simulink model "Boost_and_Two_Level_Inverter_IO"  (R2021b)
settings: Solver=ode3  StartTime=0.0  StopTime=inf  FixedStep=Ts  RelTol=1e-3
PostLoadFcn:
  | Boost_and_Two_Level_Inverter_param;
InitFcn:
  | Boost_and_Two_Level_Inverter_param;
undefined symbols (not defined in the file): arm1_g1, Boost2lvl_SFun, boost_I, Boost_PWM_Duty, Boost_PWM_Freq, boost_V, Boost_Vin, d9cbfad2d710, eHSx128_Gen4_Machines_IOConfig1, EX, fault_sw, Inv_BEMF_Ampl, Inv_PWM_CarrierFreq, Inv_PWM_ModulationIndex, Inv_PWM_Out, Inv_PWM_Phases, Inv_PWM_ShiftAngle, Ts, v1, VC707_2, vin, vsrc1, vsrc2, vsrc3
libraries: opal_lib x3, rtlab x3, rtio_opalrt_common x2, ehsSchematicEditorSourceLib x1, ehsFirmwareSelection x1
PreSaveFcn:
  | try, efsUpdateVersionAnnotation, end
settings Model: ARTEMISmethode_block_infos=$$__separator__$$  Creator=PYRobert  LastModifiedBy=ORTGRemotePC
settings SolverCC: AlgebraicLoopSolver=TrustRegion
settings DataIOCC: LimitDataPoints=on  SaveFormat=Array  SignalLoggingSaveFormat=ModelDataLogs  SaveOutput=off  SignalLogging=off  SaveTime=off  ReturnWorkspaceOutputs=off  SignalLoggingName=sigsOut
settings OptimizationCC: BlockReduction=off  OptimizeBlockIOStorage=off  BufferReuse=off  GlobalBufferReuse=off  ExpressionFolding=off  ExpressionDepthLimit=2147483647  LocalBlockOutputs=off  InitFltsAndDblsToZero=on  LifeSpan=inf  OptimizeDataStoreBuffers=off  BusAssignmentInplaceUpdate=off
settings DebuggingCC: SaveWithParameterizedLinksMsg=none  UnderspecifiedInitializationDetection=Classic  MergeDetectMultiDrivingBlocksExec=none  SignalResolutionControl=TryResolveAllWithWarning  InheritedTsInSrcMsg=none  MultiTaskDSMMsg=warning  MultiTaskCondExecSysMsg=none  ParameterOverflowMsg=none  FcnCallInpInsideContextMsg=warning  StateNameClashWarn=warning  SFUnexpectedBacktrackingDiag=warning  SFNoUnconditionalDefaultTransitionDiag=warning  SFExecutionAtInitializationDiag=none  SFMachineParentedDataDiag=warning  ArithmeticOperatorsInVariantConditions=warning
settings HardwareCC: ProdBitPerPointer=32  ProdBitPerSizeT=32  ProdBitPerPtrDiffT=32  ProdLargestAtomicFloat=None  ProdIntDivRoundTo=Undefined  ProdEndianess=Unspecified  ProdWordSize=32  ProdHWDeviceType=32-bit Generic  TargetBitPerPointer=64  TargetBitPerSizeT=64  TargetBitPerPtrDiffT=64  TargetLongLongMode=on  TargetIntDivRoundTo=Zero  TargetEndianess=LittleEndian  TargetWordSize=64  TargetHWDeviceType=MATLAB Host  ProdEqTarget=off
settings ModelReferenceCC: PropagateSignalLabelsOutOfModel=off
settings SFSimCC: SimUseLocalCustomCode=off  CustomCodeUndefinedFunction=UseInterfaceOnly
settings RTWCC: RTWUseLocalCustomCode=off
settings CodeAppCC: StateflowObjectComments=on
settings GRTTargetCC: TargetFcnLib=ansi_tfl_tmw.mat  TargetLangStandard=C89/C90 (ANSI)  CombineOutputUpdateFcns=off  GRTInterface=on
settings ConfigComp: CovMetricSettings=dw  CovSaveCumulativeToWorkspaceVar=on  CovSaveSingleToWorkspaceVar=on  CovExternalEMLEnable=off  CovSFcnEnable=off
settings SimscapeCC: SimscapeNormalizeSystem=off

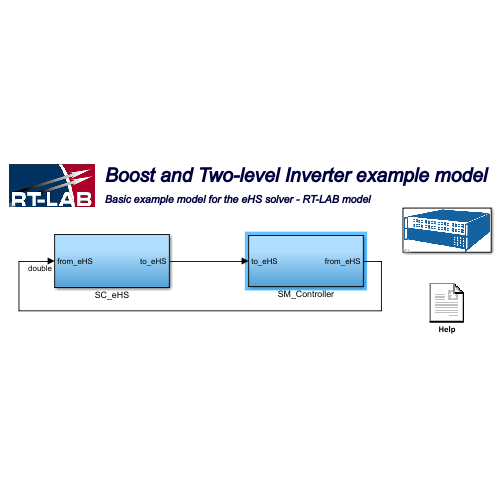
[thumbnail: Simulink's stored preview of the top-level diagram]
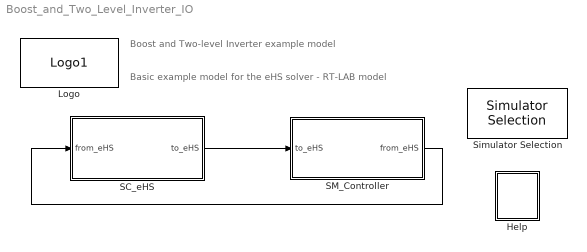
== system Boost_and_Two_Level_Inverter_IO ==
  note: Boost and Two-level Inverter example model
  note: Basic example model for the eHS solver - RT-LAB model
  Help : Subsystem  mask(OpDoc){docfile=\Docs\html\Examples\Boost-and-Two-Level-Inverter---S-Function---eHS-Gen4.html}
      mask init:
      | %patch([1,1,0,0,.8,1],[.8,0,0,1,1,.8],[.8 .8 .8]);
      | %patch([.15 .78 .78 .15 .15],[.8 .8 .83 .83 .8],[.9 .9 .9]);
      | %patch([.15 .78 .78 .15 .15],[.7 .7 .73 .73 .8],[.9 .9 .9]);
      | %patch([.15 .78 .78 .15 .15],[.6 .6 .63 .63 .6],[.9 .9 .9]);
      | %patch([.15 .78 .78 .15 .15],[.5 .5 .53 .53 .5],[.9 .9 .9]);
      | %patch([.15 .78 .78 .15 .15],[.4 .4 .43 .43 .4],[.9 .9 .9]);
      settings: OpenFcn=efsHelp_cb(gcb);
      mask Display: image(imread('opdoc.bmp'))
  Logo : opal_lib/Logo1  vide=[]
  SC_eHS : Subsystem
  SM_Controller : Subsystem
  Simulator Selection : ehsFirmwareSelection/Simulator Selection  wChassisSelection=OP5707  eHSType=SE
  wires:
  SC_eHS/1(to_eHS) -> SM_Controller/1(to_eHS)
  SM_Controller/1(from_eHS) -> SC_eHS/1(from_eHS)

== system Boost_and_Two_Level_Inverter_IO/Help ==

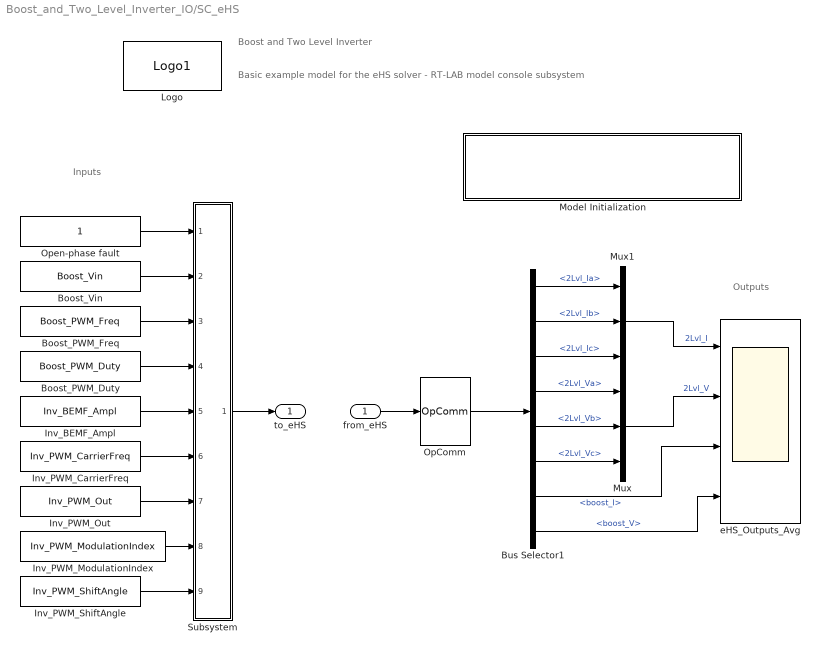
== system Boost_and_Two_Level_Inverter_IO/SC_eHS ==
  note: Inputs
  note: Outputs
  note: Boost and Two Level Inverter
  note: Basic example model for the eHS solver - RT-LAB model console subsystem
  from_eHS : Inport  OutDataTypeStr=double
  Boost_PWM_Duty : Constant  Value=Boost_PWM_Duty
  Boost_PWM_Freq : Constant  Value=Boost_PWM_Freq
  Boost_Vin : Constant  Value=Boost_Vin
  Bus Selector1 : BusSelector  OutputSignals=2Lvl_Ia,2Lvl_Ib,2Lvl_Ic,2Lvl_Va,2Lvl_Vb,2Lvl_Vc,boost_I,boost_V
  Inv_BEMF_Ampl : Constant  Value=Inv_BEMF_Ampl
  Inv_PWM_CarrierFreq : Constant  Value=Inv_PWM_CarrierFreq
  Inv_PWM_ModulationIndex : Constant  Value=Inv_PWM_ModulationIndex
  Inv_PWM_Out : Constant  Value=Inv_PWM_Out
  Inv_PWM_ShiftAngle : Constant  Value=Inv_PWM_ShiftAngle
  Logo : opal_lib/Logo1  vide=[]
  Model Initialization : Subsystem  mask(Model Functions){InitFcnX=Boost_and_Two_Level_Inverter_param;, prel=off, posl=on, inif=on, strf=off}
      mask prompts: InitFcnX "Initialisation"; prel "Preload Function"; posl "PostLoad Function"; inif "InitFcn"; strf "StartFcn"
      mask init:
      | currentBlock = gcb;
      | root = bdroot(currentBlock);
      | 
      | if ~strcmp(get_param(root,'BlockDiagramType'),'library')
      |     if prel==1
      |         set_param(root, 'PreLoadFcn', InitFcnX);
      |     else
      |         set_param(root, 'PreLoadFcn', '');
      |     end
      |     if inif==1
      |         set_param(root, 'InitFcn', InitFcnX);
      |     else
      |         set_param(root, 'InitFcn', '');
      |     end
      |     if strf==1
      |         set_param(root, 'StartFcn', InitFcnX);
      |     else
      |         set_param(root, 'StartFcn', '');
      |     end
      |     if posl==1
      |         set_param(root, 'PostLoadFcn', InitFcnX);
      |     else
      |         set_param(root, 'PostLoadFcn', '');
      |     end
      | end
      | 
      | pos = get_param(currentBlock, 'Position');
      | width = pos(3) - pos(1); height = pos(4) - pos(2);
      | txt = [ upper(root) '\n' '- InitFcn. . . . . '  get_param(root, 'InitFcn') ];
      settings: CopyFcn=set_param(gcb,'LinkStatus','none')
      mask Display: text(5, height*0.5, txt, 'horizontalAlignment', 'left', 'verticalAlignment', 'middle') ;
  Mux : Mux  Inputs=3
  Mux1 : Mux  Inputs=3
  OpComm : rtlab/OpComm  nbport=1  groupe_acq=1  subsys_rate=0  st=0  Synchronization=off  Interpolation=off  Threshold=1.0  Missed_Data=off  Sim_Time=off  Samples=off  dynSigOut=off  from_console=0  warning_done=off  writeOpCommFile=off  Offset=off
      settings: SourceProductName=RT-LAB
  Open-phase fault : Constant
  Subsystem : Subsystem
  eHS_Outputs_Avg : Scope  NumInputPorts=4
  to_eHS : Outport  VectorParamsAs1DForOutWhenUnconnected=off
  wires:
  from_eHS/1 -> OpComm/1
  Open-phase fault/1 -> Subsystem/1(In1)
  Boost_Vin/1 -> Subsystem/2(In2)
  Boost_PWM_Freq/1 -> Subsystem/3(In3)
  Boost_PWM_Duty/1 -> Subsystem/4(In4)
  Inv_BEMF_Ampl/1 -> Subsystem/5(In5)
  Inv_PWM_CarrierFreq/1 -> Subsystem/6(In7)
  Inv_PWM_Out/1 -> Subsystem/7(In8)
  Inv_PWM_ModulationIndex/1 -> Subsystem/8(In9)
  Subsystem/1(Out1) -> to_eHS/1
  OpComm/1 -> Bus Selector1/1
  Mux1/1 -> eHS_Outputs_Avg/1  "2Lvl_I"
  Inv_PWM_ShiftAngle/1 -> Subsystem/9(In10)
  Bus Selector1/1 -> Mux1/1  "<2Lvl_Ia>"
  Bus Selector1/2 -> Mux1/2  "<2Lvl_Ib>"
  Bus Selector1/4 -> Mux/1  "<2Lvl_Va>"
  Bus Selector1/6 -> Mux/3  "<2Lvl_Vc>"
  Bus Selector1/8 -> eHS_Outputs_Avg/4  "<boost_V>"
  Bus Selector1/5 -> Mux/2  "<2Lvl_Vb>"
  Bus Selector1/3 -> Mux1/3  "<2Lvl_Ic>"
  Mux/1 -> eHS_Outputs_Avg/2  "2Lvl_V"
  Bus Selector1/7 -> eHS_Outputs_Avg/3  "<boost_I>"

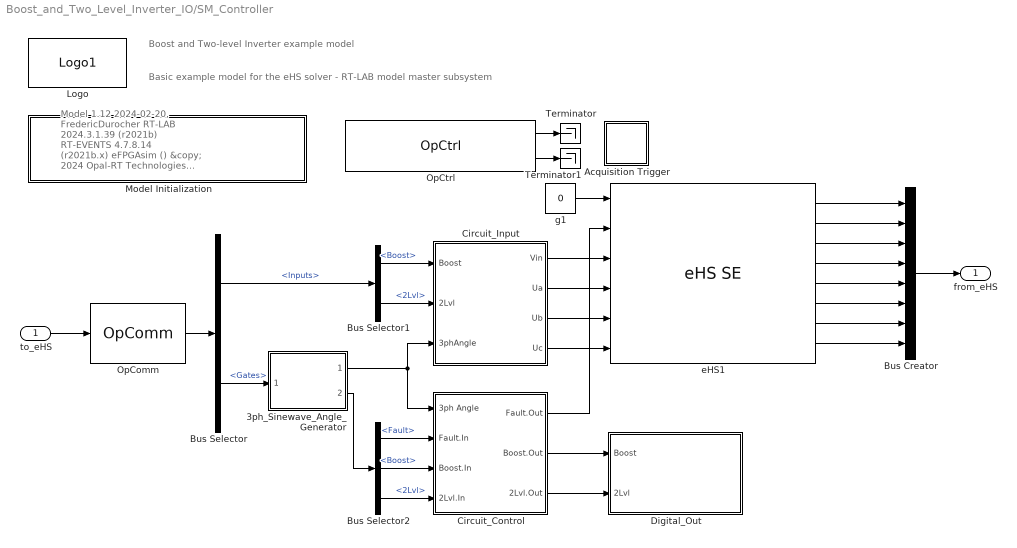
== system Boost_and_Two_Level_Inverter_IO/SM_Controller ==
  note: Model 1.12 2024-02-20, FredericDurocher
      | RT-LAB 2024.3.1.39 (r2021b)
      | RT-EVENTS 4.7.8.14 (r2021b.x)
      | eFPGAsim ()
      | &copy; 2024 Opal-RT Technologies Inc.
  note: Boost and Two-level Inverter example model
  note: Basic example model for the eHS solver - RT-LAB model master subsystem
  to_eHS : Inport
  3ph_Sinewave_Angle_Generator : Subsystem
  Acquisition Trigger : Subsystem
  Bus Creator : BusCreator  Inputs=8
  Bus Selector : BusSelector  OutputSignals=Inputs,Gates
  Bus Selector1 : BusSelector  OutputSignals=Boost,2Lvl
  Bus Selector2 : BusSelector  OutputSignals=Fault,Boost,2Lvl
  Circuit_Control : Subsystem
  Circuit_Input : Subsystem
  Digital_Out : Subsystem
  Logo : opal_lib/Logo1  vide=[]
  Model Initialization : Subsystem  mask(Model Functions){InitFcnX=Boost_and_Two_Level_Inverter_param;, prel=off, posl=on, inif=on, strf=off}
      mask prompts: InitFcnX "Initialisation"; prel "Preload Function"; posl "PostLoad Function"; inif "InitFcn"; strf "StartFcn"
      mask init: same as Boost_and_Two_Level_Inverter_IO/SC_eHS/Model Initialization
      settings: CopyFcn=set_param(gcb,'LinkStatus','none')
      mask Display: text(5, height*0.5, txt, 'horizontalAlignment', 'left', 'verticalAlignment', 'middle') ;
  OpComm : rtlab/OpComm  nbport=1  groupe_acq=1  subsys_rate=0  st=0  Synchronization=on  Interpolation=on  Threshold=1.0  Missed_Data=off  Sim_Time=off  Samples=off  dynSigOut=off  from_console=1  warning_done=off  writeOpCommFile=off  Offset=off
      settings: SourceProductName=RT-LAB
  OpCtrl : rtio_opalrt_common/OpCtrl  CtrlName='OpCtrl'  boardid=0  BitstreamFilename=VC707_2-EX-0001-3_5_0_817-eHSx128_Gen4_Machines_IOConfig1-35-60.bin  numconfig=-1  mode=Master  externalClock=off  decimRtsi=0  calibIO=off  SampleTime=0  loadinport=-1  BoardType=VC707  SecondaryPresent=off  sync_type=Audio  scope_enable=off  fsdFileName=VC707_2-EX-0001-3_4_0_820-eHSx128_Gen4_Machines_IOConfig1-35-4E.fsd  mismatch_disable=off
      settings: SourceProductName=RT-LAB I/O
  Terminator : Terminator
  Terminator1 : Terminator
  eHS1 : ehsSchematicEditorSourceLib/eHS SE  opCtrlName='OpCtrl'  modelName=Boost2lvl_SFun - v1  modelUuid=4f5454b4-827f-4460-8912-d9cbfad2d710  modelDisplayName=Boost2lvl_SFun  lastLoadedModelText=Circuit loaded on 04-Nov-2024 12:07:51  lastLoadedModelName=Boost2lvl_SFun - v1  lastLoadedModelUuid=4f5454b4-827f-4460-8912-d9cbfad2d710  lastLoadedModelDisplayName=Boost2lvl_SFun - v1  triggerUpdate=off  timeStepInfo=Time Step: 230 ns (Min: 230 ns)  inputPins=arm1_g1,fault_sw,vin,vsrc1,vsrc2,vsrc3  outputPins=2Lvl_Ia,2Lvl_Ib,2Lvl_Ic,2Lvl_Va,2Lvl_Vb,2Lvl_Vc,boost_I,boost_V  loadPassed=1  firmwareName=VC707_2-EX-0001-3_5_0_817-eHSx128_Gen4_Machines_IOConfig1-35-60.bin  autoConfigureFirmware=on  driverType=SFUN  ehsEffectiveLicense=x128
  g1 : Constant  Value=0
  from_eHS : Outport  VectorParamsAs1DForOutWhenUnconnected=off
  wires:
  to_eHS/1 -> OpComm/1
  OpComm/1 -> Bus Selector/1
  Circuit_Control/2(Boost.Out) -> Digital_Out/1(Boost)
  Circuit_Control/3(2Lvl.Out) -> Digital_Out/2(2Lvl)
  Bus Selector1/1 -> Circuit_Input/1(Boost)  "<Boost>"
  Bus Selector1/2 -> Circuit_Input/2(2Lvl)  "<2Lvl>"
  Bus Selector/1 -> Bus Selector1/1  "<Inputs>"
  Bus Selector/2 -> 3ph_Sinewave_Angle_Generator/1(Params.In)  "<Gates>"
  Bus Selector2/3 -> Circuit_Control/4(2Lvl.In)  "<2Lvl>"
  Bus Selector2/2 -> Circuit_Control/3(Boost.In)  "<Boost>"
  Bus Selector2/1 -> Circuit_Control/2(Fault.In)  "<Fault>"
  3ph_Sinewave_Angle_Generator/2(Params.Out) -> Bus Selector2/1
  3ph_Sinewave_Angle_Generator/1(3ph_Angle) -> Circuit_Input/3(3phAngle), Circuit_Control/1(3ph Angle)
  Bus Creator/1 -> from_eHS/1
  Circuit_Control/1(Fault.Out) -> eHS1/2
  Circuit_Input/1(Vin) -> eHS1/3
  Circuit_Input/2(Ua) -> eHS1/4
  Circuit_Input/3(Ub) -> eHS1/5
  Circuit_Input/4(Uc) -> eHS1/6
  eHS1/2 -> Bus Creator/2
  eHS1/3 -> Bus Creator/3
  eHS1/4 -> Bus Creator/4
  eHS1/5 -> Bus Creator/5
  eHS1/6 -> Bus Creator/6
  eHS1/7 -> Bus Creator/7
  eHS1/8 -> Bus Creator/8
  g1/1 -> eHS1/1
  OpCtrl/1 -> Terminator/1
  OpCtrl/2 -> Terminator1/1
  eHS1/1 -> Bus Creator/1

== system Boost_and_Two_Level_Inverter_IO/SC_eHS/Model Initialization ==

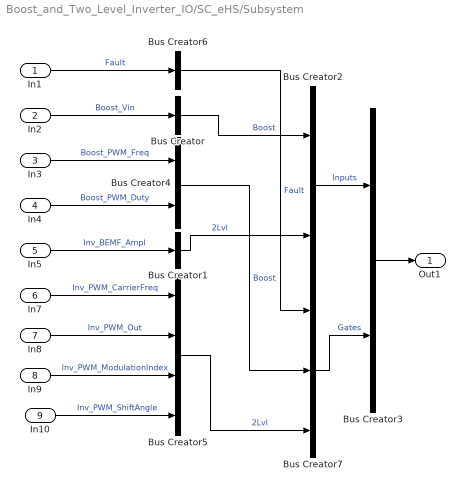
== system Boost_and_Two_Level_Inverter_IO/SC_eHS/Subsystem ==
  In1 : Inport
  In2 : Inport  Port=2
  In3 : Inport  Port=3
  In4 : Inport  Port=4
  In5 : Inport  Port=5
  In7 : Inport  Port=6
  In8 : Inport  Port=7
  In9 : Inport  Port=8
  In10 : Inport  Port=9
  Bus Creator : BusCreator  Inputs=1
  Bus Creator1 : BusCreator  Inputs=1
  Bus Creator2 : BusCreator  Inputs=2
  Bus Creator3 : BusCreator  Inputs=2
  Bus Creator4 : BusCreator  Inputs=2
  Bus Creator5 : BusCreator  Inputs=4
  Bus Creator6 : BusCreator  Inputs=1
  Bus Creator7 : BusCreator  Inputs=3
  Out1 : Outport  VectorParamsAs1DForOutWhenUnconnected=off
  wires:
  In4/1 -> Bus Creator4/2  "Boost_PWM_Duty"
  Bus Creator2/1 -> Bus Creator3/1  "Inputs"
  Bus Creator1/1 -> Bus Creator2/2  "2Lvl"
  In8/1 -> Bus Creator5/2  "Inv_PWM_Out"
  In5/1 -> Bus Creator1/1  "Inv_BEMF_Ampl"
  In1/1 -> Bus Creator6/1  "Fault"
  In2/1 -> Bus Creator/1  "Boost_Vin"
  Bus Creator/1 -> Bus Creator2/1  "Boost"
  Bus Creator7/1 -> Bus Creator3/2  "Gates"
  In9/1 -> Bus Creator5/3  "Inv_PWM_ModulationIndex"
  Bus Creator4/1 -> Bus Creator7/2  "Boost"
  In3/1 -> Bus Creator4/1  "Boost_PWM_Freq"
  In7/1 -> Bus Creator5/1  "Inv_PWM_CarrierFreq"
  Bus Creator3/1 -> Out1/1
  Bus Creator6/1 -> Bus Creator7/1  "Fault"
  Bus Creator5/1 -> Bus Creator7/3  "2Lvl"
  In10/1 -> Bus Creator5/4  "Inv_PWM_ShiftAngle"

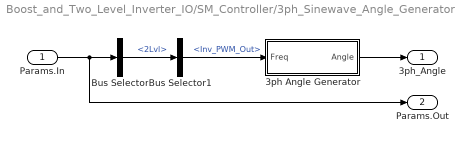
== system Boost_and_Two_Level_Inverter_IO/SM_Controller/3ph_Sinewave_Angle_Generator ==
  Params.In : Inport
  3ph Angle Generator : Subsystem
  Bus Selector : BusSelector  OutputSignals=2Lvl
  Bus Selector1 : BusSelector  OutputSignals=Inv_PWM_Out
  3ph_Angle : Outport  VectorParamsAs1DForOutWhenUnconnected=off
  Params.Out : Outport  Port=2  VectorParamsAs1DForOutWhenUnconnected=off
  wires:
  Params.In/1 -> Params.Out/1, Bus Selector/1
  Bus Selector/1 -> Bus Selector1/1  "<2Lvl>"
  Bus Selector1/1 -> 3ph Angle Generator/1(Freq)  "<Inv_PWM_Out>"
  3ph Angle Generator/1(Angle) -> 3ph_Angle/1

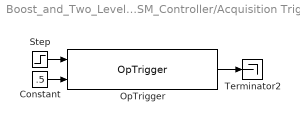
== system Boost_and_Two_Level_Inverter_IO/SM_Controller/Acquisition Trigger ==
  Constant : Constant  Value=.5
  OpTrigger : rtlab/DataLogging/OpTrigger  Trig_Type=TRIGGER SIGNAL >= TRIGGER LEVEL  Trig_Offset=0  Acq_Group=1
      settings: SourceProductName=RT-LAB
  Step : Step  Time=0.5  SampleTime=Ts
  Terminator2 : Terminator
  wires:
  Constant/1 -> OpTrigger/2
  Step/1 -> OpTrigger/1
  OpTrigger/1 -> Terminator2/1

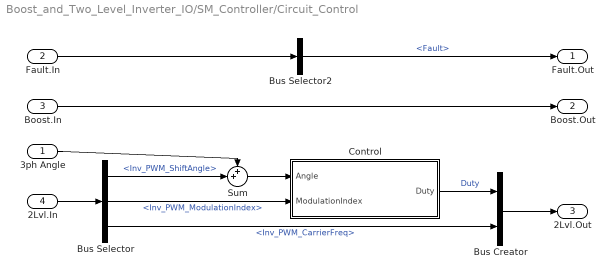
== system Boost_and_Two_Level_Inverter_IO/SM_Controller/Circuit_Control ==
  3ph Angle : Inport
  Fault.In : Inport  Port=2
  Boost.In : Inport  Port=3
  2Lvl.In : Inport  Port=4
  Bus Creator : BusCreator  Inputs=2
  Bus Selector : BusSelector  OutputSignals=Inv_PWM_ShiftAngle,Inv_PWM_ModulationIndex,Inv_PWM_CarrierFreq
  Bus Selector2 : BusSelector  OutputSignals=Fault
  Control : Subsystem
  Sum : Sum  Inputs=++|
  Fault.Out : Outport  VectorParamsAs1DForOutWhenUnconnected=off
  Boost.Out : Outport  Port=2  VectorParamsAs1DForOutWhenUnconnected=off
  2Lvl.Out : Outport  Port=3  VectorParamsAs1DForOutWhenUnconnected=off
  wires:
  Boost.In/1 -> Boost.Out/1
  Bus Creator/1 -> 2Lvl.Out/1
  2Lvl.In/1 -> Bus Selector/1
  Fault.In/1 -> Bus Selector2/1
  Bus Selector2/1 -> Fault.Out/1  "<Fault>"
  Bus Selector/2 -> Control/2(ModulationIndex)  "<Inv_PWM_ModulationIndex>"
  Control/1(Duty) -> Bus Creator/1  "Duty"
  Bus Selector/3 -> Bus Creator/2  "<Inv_PWM_CarrierFreq>"
  Sum/1 -> Control/1(Angle)
  Bus Selector/1 -> Sum/2  "<Inv_PWM_ShiftAngle>"
  3ph Angle/1 -> Sum/1

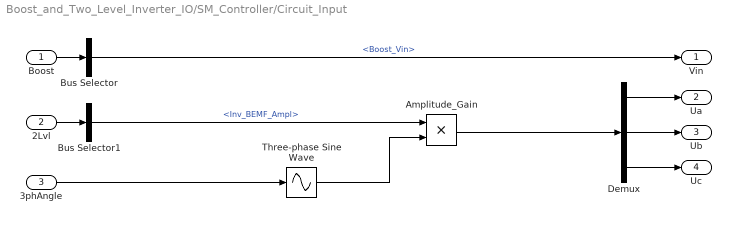
== system Boost_and_Two_Level_Inverter_IO/SM_Controller/Circuit_Input ==
  Boost : Inport
  2Lvl : Inport  Port=2
  3phAngle : Inport  Port=3
  Amplitude_Gain : Product  RndMeth=Zero
  Bus Selector : BusSelector  OutputSignals=Boost_Vin
  Bus Selector1 : BusSelector  OutputSignals=Inv_BEMF_Ampl
  Demux : Demux  Outputs=3
  Three-phase Sine Wave : Sin  TimeSource=Use external signal  Phase=Inv_PWM_Phases
  Vin : Outport  VectorParamsAs1DForOutWhenUnconnected=off
  Ua : Outport  Port=2  VectorParamsAs1DForOutWhenUnconnected=off
  Ub : Outport  Port=3  VectorParamsAs1DForOutWhenUnconnected=off
  Uc : Outport  Port=4  VectorParamsAs1DForOutWhenUnconnected=off
  wires:
  Boost/1 -> Bus Selector/1
  Bus Selector/1 -> Vin/1  "<Boost_Vin>"
  2Lvl/1 -> Bus Selector1/1
  Demux/1 -> Ua/1
  Demux/2 -> Ub/1
  Demux/3 -> Uc/1
  Bus Selector1/1 -> Amplitude_Gain/1  "<Inv_BEMF_Ampl>"
  Amplitude_Gain/1 -> Demux/1
  Three-phase Sine Wave/1 -> Amplitude_Gain/2
  3phAngle/1 -> Three-phase Sine Wave/1

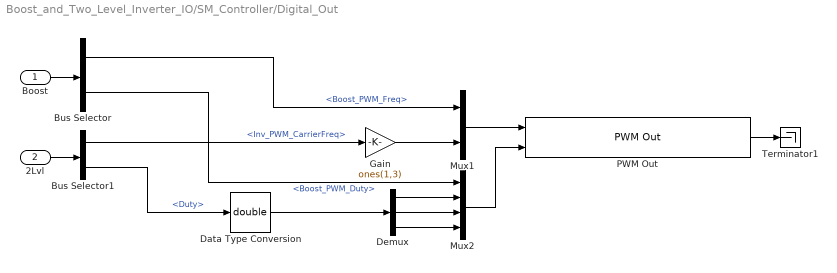
== system Boost_and_Two_Level_Inverter_IO/SM_Controller/Digital_Out ==
  Boost : Inport
  2Lvl : Inport  Port=2
  Bus Selector : BusSelector  OutputSignals=Boost_PWM_Freq,Boost_PWM_Duty
  Bus Selector1 : BusSelector  OutputSignals=Inv_PWM_CarrierFreq,Duty
  Data Type Conversion : DataTypeConversion  OutDataTypeStr=double
  Demux : Demux  Outputs=3
  Gain : Gain  Gain=ones(1,3)
  Mux1 : Mux  Inputs=2
  Mux2 : Mux
  PWM Out : rtio_opalrt_common/PWM Out  CtrlName='OpCtrl'  portNb=11  FcnNos=Slot 0 Module X Subsection 0  size=0  maxcount=0  count=4  polarity=Active High  symMode=Asymmetric  rtPhaseDeadTimeEnabled=on  allowDisablingChannel=off  complementary=off  rtDeadTimeEnabled=off  deadTime=[0 0 0 0]  numchan=4  loadnb=-64  rtPhaseShiftEnabled=off  initphase=[0 0 0 0]
      settings: AttributesFormatString=%<CtrlName>  SourceProductName=RT-LAB I/O
  Terminator1 : Terminator
  wires:
  Bus Selector/1 -> Mux1/1  "<Boost_PWM_Freq>"
  Bus Selector/2 -> Mux2/1  "<Boost_PWM_Duty>"
  Boost/1 -> Bus Selector/1
  2Lvl/1 -> Bus Selector1/1
  Bus Selector1/2 -> Data Type Conversion/1  "<Duty>"
  Data Type Conversion/1 -> Demux/1
  Bus Selector1/1 -> Gain/1  "<Inv_PWM_CarrierFreq>"
  Mux1/1 -> PWM Out/1
  Gain/1 -> Mux1/2
  Demux/2 -> Mux2/3
  Demux/1 -> Mux2/2
  Demux/3 -> Mux2/4
  Mux2/1 -> PWM Out/2
  PWM Out/1 -> Terminator1/1

== system Boost_and_Two_Level_Inverter_IO/SM_Controller/Model Initialization ==

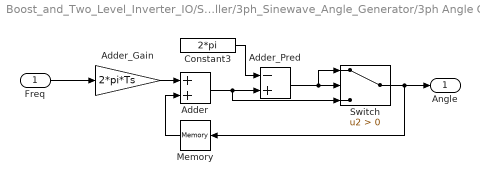
== system Boost_and_Two_Level_Inverter_IO/SM_Controller/3ph_Sinewave_Angle_Generator/3ph Angle Generator ==
  Freq : Inport
  Adder : Sum
  Adder_Gain : Gain  Gain=2*pi*Ts  OutDataTypeStr=double
  Adder_Pred : Sum  Inputs=-+
  Constant3 : Constant  Value=2*pi  OutDataTypeStr=double
  Memory : Memory  InheritSampleTime=on
  Switch : Switch  Criteria=u2 > Threshold
  Angle : Outport  VectorParamsAs1DForOutWhenUnconnected=off
  wires:
  Memory/1 -> Adder/2
  Freq/1 -> Adder_Gain/1
  Adder/1 -> Switch/3, Adder_Pred/2
  Adder_Gain/1 -> Adder/1
  Constant3/1 -> Adder_Pred/1
  Switch/1 -> Angle/1, Memory/1
  Adder_Pred/1 -> Switch/2, Switch/1

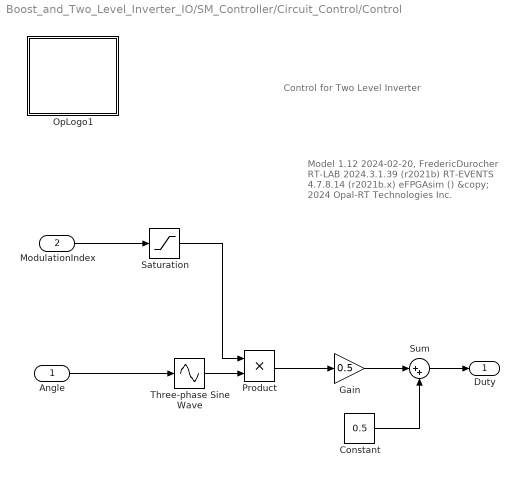
== system Boost_and_Two_Level_Inverter_IO/SM_Controller/Circuit_Control/Control ==
  note: Control for Two Level Inverter
  note: Model 1.12 2024-02-20, FredericDurocher
      | RT-LAB 2024.3.1.39 (r2021b)
      | RT-EVENTS 4.7.8.14 (r2021b.x)
      | eFPGAsim ()
      | &copy; 2024 Opal-RT Technologies Inc.
  Angle : Inport
  ModulationIndex : Inport  Port=2
  Constant : Constant  Value=0.5
  Gain : Gain  Gain=0.5
  OpLogo1 : Subsystem
  Product : Product  RndMeth=Zero
  Saturation : Saturate  UpperLimit=0.95  LowerLimit=0.05  OutDataTypeStr=Inherit: Inherit via back propagation
  Sum : Sum  Inputs=|++
  Three-phase Sine Wave : Sin  TimeSource=Use external signal  Phase=Inv_PWM_Phases
  Duty : Outport  VectorParamsAs1DForOutWhenUnconnected=off
  wires:
  ModulationIndex/1 -> Saturation/1
  Saturation/1 -> Product/1
  Product/1 -> Gain/1
  Gain/1 -> Sum/1
  Sum/1 -> Duty/1
  Constant/1 -> Sum/2
  Angle/1 -> Three-phase Sine Wave/1
  Three-phase Sine Wave/1 -> Product/2

== system Boost_and_Two_Level_Inverter_IO/SM_Controller/Circuit_Control/Control/OpLogo1 ==
